simulink model "epidemia"  (Simulink 7.2)
settings: Solver=ode45  StartTime=0.0  StopTime=60  FixedStep=1e-3  RelTol=1e-5  AbsTol=1e-6
values from neighbouring files (symbols this model uses):
  mu = dmu*mun    [ms_epidemia.m]
  N0 = sum(x0)    [ms_epidemia.m]
  ni = dni*nin    [ms_epidemia.m]
  R0 = PieGuariti + PieIsolamento + PieDeceduti + 200    [ms_epidemia.m]
  x0 = [S0 E0 I0 R0]'    [ms_epidemia.m]
libraries: simulink_extras x2
settings Model: Creator=prof. G. Celentano  LastModifiedBy=prof. G. Celentano
settings DebuggingCC: SolverPrmCheckMsg=none

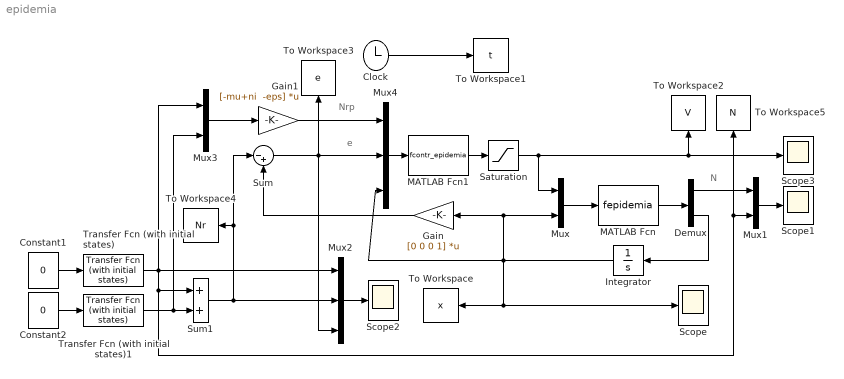
== system epidemia ==
  note: e
  note: Nrp
  note: N
  Clock : Clock
      settings: Decimation=10
  Constant1 : Constant  Value=0  OutDataType=sfix(16)  OutScaling=2^0
  Constant2 : Constant  Value=0  OutDataType=sfix(16)  OutScaling=2^0
  Demux : Demux  Outputs=[1 4]
  Gain : Gain  Orientation=left  Gain=[0 0 0 1]  Multiplication=Matrix(K*u)  ParameterDataType=sfix(16)  ParameterScaling=2^0  OutDataType=sfix(16)  OutScaling=2^0
  Gain1 : Gain  Gain="[-mu+ni  -eps]"  Multiplication=Matrix(K*u)  ParameterDataType=sfix(16)  ParameterScaling=2^0  OutDataType=sfix(16)  OutScaling=2^0
  Integrator : Integrator  Orientation=left  InitialCondition=x0
  MATLAB Fcn : MATLABFcn  MATLABFcn=fepidemia  OutputDimensions=5
  MATLAB Fcn1 : MATLABFcn  MATLABFcn=fcontr_epidemia  OutputDimensions=1
  Mux : Mux  Inputs=[1 4]
  Mux1 : Mux  Inputs=2
  Mux2 : Mux  Inputs=3
  Mux3 : Mux  Inputs=2
  Mux4 : Mux  Inputs=[1 1 4]
  Saturation : Saturate  UpperLimit=1  LowerLimit=0  OutDataType=sfix(16)  OutScaling=2^0
  Scope{,1..3} (4 alike) : Scope
      Scope settings: TimeRange=50  YMin=0  YMax=1400
      Scope1 settings: YMin=-1750  YMax=1000
      Scope2 settings: TimeRange=50  YMin=-2000000  YMax=1000000  SaveName=ScopeData2
      Scope3 settings: YMin=-1750  YMax=1000  SaveName=ScopeData3
  Sum : Sum  Inputs=|-+  OutDataType=sfix(16)  OutScaling=2^0
  Sum1 : Sum  OutDataType=sfix(16)  OutScaling=2^0
  To Workspace : ToWorkspace  VariableName=x  SampleTime=-1  SaveFormat=Array
  To Workspace1 : ToWorkspace  VariableName=t  SampleTime=-1  SaveFormat=Array
  To Workspace2 : ToWorkspace  VariableName=V  SampleTime=-1  SaveFormat=Array
      settings: Orientation=up
  To Workspace3 : ToWorkspace  VariableName=e  SampleTime=-1  SaveFormat=Array
      settings: Orientation=up
  To Workspace4 : ToWorkspace  VariableName=Nr  SampleTime=-1  SaveFormat=Array
  To Workspace5 : ToWorkspace  VariableName=N  SampleTime=-1  SaveFormat=Array
      settings: Orientation=up
  Transfer Fcn (with initial states) : simulink_extras/Additional Linear/Transfer Fcn (with initial states)  SystemSampleTime=-1  N=1  D=[1 mu-ni]  X0=N0
  Transfer Fcn (with initial states)1 : simulink_extras/Additional Linear/Transfer Fcn (with initial states)  SystemSampleTime=-1  N=1  D=[1 eps]  X0=(R0-N0)
  wires:
  MATLAB Fcn/1 -> Demux/1
  Demux/2 -> Integrator/1
  Mux/1 -> MATLAB Fcn/1
  MATLAB Fcn1/1 -> Saturation/1
  Integrator/1 -> Scope/1, To Workspace/1, Mux/2, Gain/1, Mux4/3
  Mux1/1 -> Scope1/1
  Constant1/1 -> Transfer Fcn (with initial states)/1
  Constant2/1 -> Transfer Fcn (with initial states)1/1
  Transfer Fcn (with initial states)/1 -> Mux2/1, Mux3/1, Sum1/1, Mux1/2, To Workspace5/1
  Transfer Fcn (with initial states)1/1 -> Sum1/2, Mux3/2
  Sum1/1 -> Mux2/2, Sum/1, To Workspace4/1
  Mux2/1 -> Scope2/1
  Clock/1 -> To Workspace1/1
  Gain/1 -> Sum/2
  Mux3/1 -> Gain1/1
  Mux4/1 -> MATLAB Fcn1/1
  Gain1/1 -> Mux4/1
  Sum/1 -> Mux2/3, Mux4/2, To Workspace3/1
  Saturation/1 -> Mux/1, To Workspace2/1, Scope3/1
  Demux/1 -> Mux1/1
